simulink model "ask"  (R2018b)
settings: Solver=VariableStepAuto  StartTime=0.0  StopTime=100.0  RelTol=1e-3
libraries: dsparch4 x2, commrandsrc3 x1
settings Model: Creator=86138  LastModifiedBy=86138

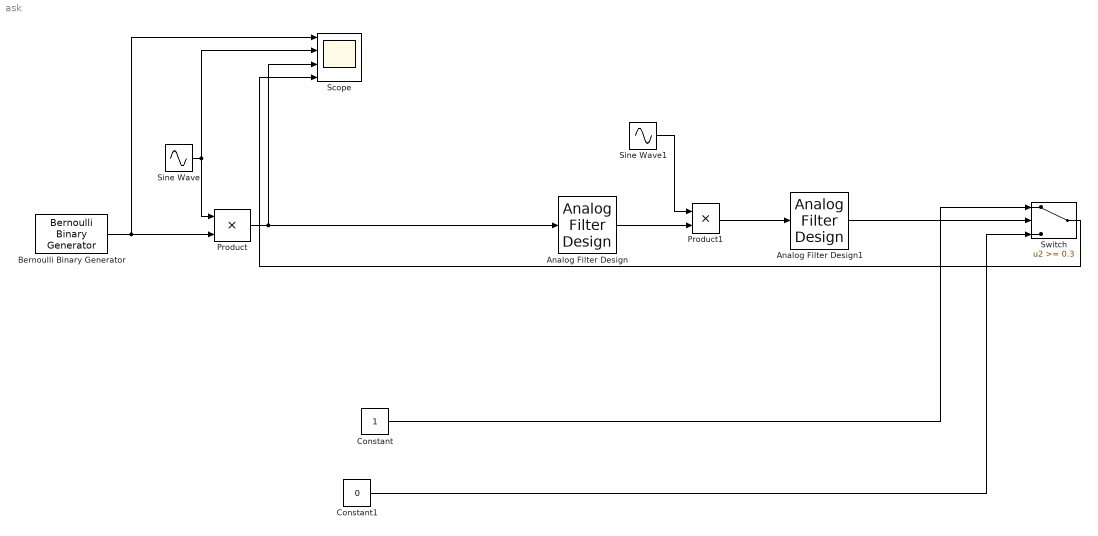
== system ask ==
  Analog Filter Design : dsparch4/Analog Filter Design  method=Butterworth  filttype=Bandpass  N=2  Wlo=4*pi  Whi=10*pi  Rp=2  Rs=40
  Analog Filter Design1 : dsparch4/Analog Filter Design  method=Butterworth  filttype=Lowpass  N=2  Wlo=6*pi  Whi=80  Rp=2  Rs=40
  Bernoulli Binary Generator : commrandsrc3/Bernoulli Binary Generator  ProbabilityOfZero=0.5  SeedSource=Auto  Seed=0  SampleTime=1  SamplesPerFrame=1  OutputDataType=double  SimulateUsing=Interpreted execution
  Constant : Constant
  Constant1 : Constant  Value=0
  Product : Product
  Product1 : Product
  Scope : Scope  NumInputPorts=4
  Sine Wave : Sin  Frequency=6*pi  SampleTime=0
  Sine Wave1 : Sin  Frequency=6*pi  SampleTime=0
  Switch : Switch  Threshold=0.3
  wires:
  Bernoulli Binary Generator/1 -> Scope/1, Product/2
  Sine Wave/1 -> Product/1, Scope/2
  Product/1 -> Analog Filter Design/1, Scope/3
  Product1/1 -> Analog Filter Design1/1
  Analog Filter Design/1 -> Product1/2
  Sine Wave1/1 -> Product1/1
  Analog Filter Design1/1 -> Switch/2
  Constant/1 -> Switch/1
  Constant1/1 -> Switch/3
  Switch/1 -> Scope/4
